simulink model "Flux_Estimator"  (R2014a)
settings: Solver=ode23tb  StartTime=0.0  StopTime=1  MaxStep=50e-6  RelTol=1e-3
libraries: powerlib x10, powerlib_meascontrol x2
settings Model: Creator=ninad gaikawad  LastModifiedBy=ninad gaikawad
settings SolverCC: ZeroCrossControl=EnableAll  ZeroCrossAlgorithm=Adaptive  AutoInsertRateTranBlk=on
settings DebuggingCC: AlgebraicLoopMsg=error

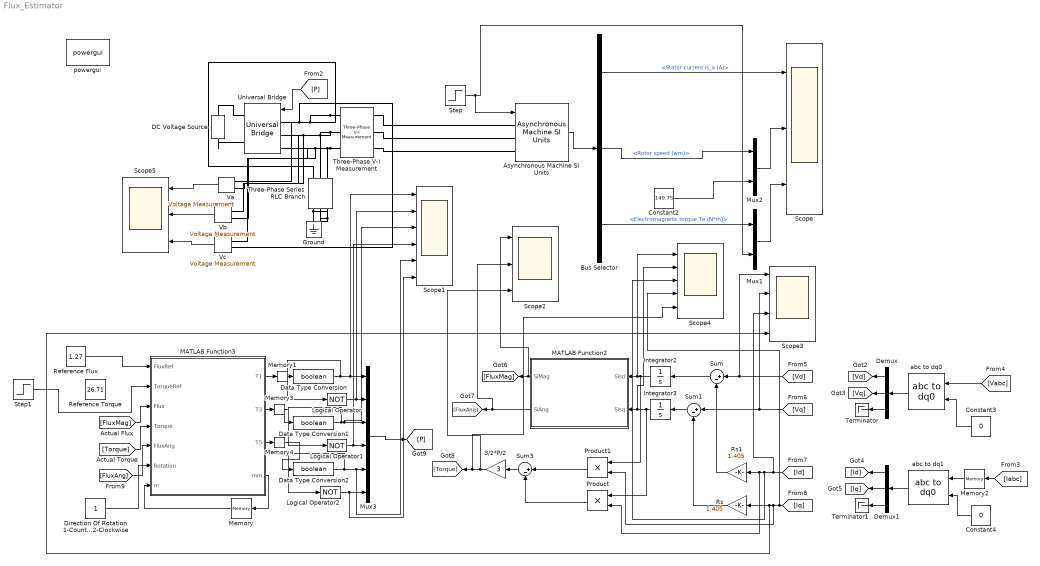
== system Flux_Estimator ==
  3/2*P/2 : Gain  Gain=3
  Asynchronous Machine SI Units : powerlib/Machines/Asynchronous Machine SI Units  PresetModel="15:  5.4 HP (4KW)   400 V  50Hz 1430 RPM"  MechanicalLoad=Torque Tm  ShowDetailedParameters=on  RotorType=Squirrel-cage  ReferenceFrame=Rotor  Units=SI  MeasurementBus=off  NominalParameters=[4000 400 50]  Stator=[1.405 0.005839]  Rotor=[1.395 0.005839]  Cage1=[ 0.022 0.226/377]  Cage2=[ 0.022 0.226/377]  Lm=0.1722  Mechanical=[0.0131 0.002985 2]  PolePairs=2  InitialConditions=[1 0 0 0 0 0 0 0]  SimulateSaturation=off  Saturation=[14.03593122, 27.81365428, 53.79336849, 72.68890987, 97.98006896, 148.6815601, 215.7428561, 302.9841135, 420.4778367 ; 230, 322, 414, 460, 506, 552, 598, 644, 690]  LoadFlowParameters=1492000  TsPowergui=0  TsBlock=-1  IterativeModel=Trapezoidal non iterative  Pmec=0
  Bus Selector : BusSelector  OutputSignals=Stator measurements.Stator current is_a (A),Mechanical.Rotor speed (wm),Mechanical.Electromagnetic torque Te (N*m)
  Constant2 : Constant  Value=149.75
  Constant3 : Constant  Value=0
  Constant4 : Constant  Value=0
  DC Voltage Source : powerlib/Electrical Sources/DC Voltage Source  Amplitude=565.7  Measurements=None
  Data Type Conversion : DataTypeConversion  OutDataTypeStr=boolean
  Data Type Conversion1 : DataTypeConversion  OutDataTypeStr=boolean
  Data Type Conversion2 : DataTypeConversion  OutDataTypeStr=boolean
  Demux : Demux  Outputs=3
  Demux1 : Demux  Outputs=3
  Direction Of Rotation 1-CounterClockwise 2-Clockwise : Constant
  Ground : powerlib/Elements/Ground  LConnTagsString=a
  Integrator2 : Integrator
  Integrator3 : Integrator
  Logical Operator : Logic  Operator=NOT  AllPortsSameDT=off  OutDataTypeStr=boolean
  Logical Operator1 : Logic  Operator=NOT  AllPortsSameDT=off  OutDataTypeStr=boolean
  Logical Operator2 : Logic  Operator=NOT  AllPortsSameDT=off  OutDataTypeStr=boolean
  MATLAB Function2 : MATLAB Function  TreatAsAtomicUnit=on
  MATLAB Function3 : MATLAB Function  TreatAsAtomicUnit=on
  Memory : Memory  X0=1
  Memory1 : Memory  X0=1
  Memory2 : Memory  X0=1
  Memory3 : Memory
  Memory4 : Memory
  Mux1 : Mux  Inputs=2
  Mux2 : Mux  Inputs=2
  Mux3 : Mux  Inputs=6
  Product : Product
  Product1 : Product
  Reference Flux : Constant  Value=1.27
  Reference Torque : Constant  Value=26.71
  Rs : Gain  Gain=1.405
  Rs1 : Gain  Gain=1.405
  Scope : Scope  NumInputPorts=3
      settings: YMin=-0.31398~-350~0  YMax=-0.284078~150~0.00225
  Scope1 : Scope  NumInputPorts=6
      settings: YMin=-5~-5~-5~-5~-5~-5  YMax=5~5~5~5~5~5
  Scope2 : Scope  NumInputPorts=3
      settings: YMin=-5~-5~-5  YMax=5~5~5  SaveName=ScopeData2
  Scope3 : Scope  NumInputPorts=4
      settings: TimeRange=10  YMin=-400~-400~-266.8~-1  YMax=200~400~-266.35~0.5  SaveName=ScopeData3
  Scope4 : Scope  NumInputPorts=5
      settings: YMin=-5~-5~-5~-5~-5  YMax=5~5~5~5~5  SaveName=ScopeData4
  Scope5 : Scope  NumInputPorts=3
      settings: YMin=-5~-5~-5  YMax=5~5~5  SaveName=ScopeData5
  Step : Step  Time=0.5  After=26.71  SampleTime=0
  Step1 : Step  Time=0.5  After=26.71  SampleTime=0
  Sum : Sum  Inputs=|+-
  Sum1 : Sum  Inputs=|+-
  Sum3 : Sum  Inputs=|+-
  Terminator : Terminator
  Terminator1 : Terminator
  Three-Phase Series RLC Branch : powerlib/Elements/Three-Phase Series RLC Branch  LConnTagsString=A|B|C  RConnTagsString=A|B|C  BranchType=R  Resistance=1e6  Inductance=1e-3  Capacitance=1e-6  Measurements=None
  Three-Phase V-I Measurement : powerlib/Measurements/Three-Phase V-I Measurement  VoltageMeasurement=phase-to-ground  SetLabelV=on  LabelV=Vabc  Vpu=off  VpuLL=off  CurrentMeasurement=yes  SetLabelI=on  LabelI=Iabc  Ipu=off  Pbase=100e6  Vbase=500e3  OutputType=Complex  PhasorSimulation=off  PSBequivalent=0
  Universal Bridge : powerlib/Power Electronics/Universal Bridge  Arms=3  SnubberResistance=1e5  SnubberCapacitance=inf  Device=IGBT / Diodes  Ron=1e-3  Lon=0  ForwardVoltages="[  0  0  ]"  ForwardVoltage=0  GTOparameters=[ 10e-6 , 20e-6 ]  IGBTparameters=[ 1e-6 , 2e-6 ]  Measurements=None  Measurements_2=None  converterType=Rectifier
  Va : powerlib/Measurements/Voltage Measurement  PhasorSimulation=off  OutputType=Complex  PSBequivalent=0
  Vb : powerlib/Measurements/Voltage Measurement  PhasorSimulation=off  OutputType=Complex  PSBequivalent=0
  Vc : powerlib/Measurements/Voltage Measurement  PhasorSimulation=off  OutputType=Complex  PSBequivalent=0
  abc to dq0 : powerlib_meascontrol/Transformations/abc to dq0  Alignment=Aligned with phase A axis
  abc to dq1 : powerlib_meascontrol/Transformations/abc to dq0  Alignment=Aligned with phase A axis
  powergui : powerlib/powergui  Priority=1  SimulationMode=Continuous  SolverType=Tustin  SampleTime=50e-6  frequency=60  SPID=off  DisableSnubberDevices=off  DisableRonSwitches=off  DisableVfSwitches=off  SwTol=0  Interpol=off  DisplayEquations=off  Ts=0  methode=off  frequencyindice=50  Pbase=100e6  ErrMax=1e-4  Iterations=50  UnitsV=kV  UnitsW=MW  FunctionMessages=off  echomessages=off  HookPort=off  EnableUseOfTLC=off  x0status=blocks  RestoreLinks=warning  ResistiveCurrentMeasurement=off  Frange=[0:2:500]  Ylog=off  Xlog=on  ShowGrid=off  save=off  variable=ZData  structure=0  ZoomFFT=off  StartTime=0.0  cycles=1  DisplayStyle=1  fundamental=60  FreqAxis=off  MaxFrequency=1000  frequencyindicesteady=1  RmsSteady=1  display=off
  wires:
  Asynchronous Machine SI Units/1 -> Bus Selector/1
  Mux1/1 -> Scope/3
  Mux2/1 -> Scope/2
  [P] -> Universal Bridge/1
  Bus Selector/1 -> Scope/1  "<Stator current is_a (A)>"
  Bus Selector/2 -> Mux2/1  "<Rotor speed (wm)>"
  Bus Selector/3 -> Mux1/1  "<Electromagnetic torque Te (N*m)>"
  Constant2/1 -> Mux2/2
  Constant3/1 -> abc to dq0/2
  Constant4/1 -> abc to dq1/2
  abc to dq0/1 -> Demux/1
  abc to dq1/1 -> Demux1/1
  Demux1/3 -> Terminator1/1
  Demux/3 -> Terminator/1
  Demux1/2 -> [Iq]
  Demux1/1 -> [Id]
  Demux/1 -> [Vd]
  Demux/2 -> [Vq]
  [Id] -> Scope3/3, Scope4/3, Product/2, Rs1/1
  [Iq] -> Scope4/4, Product1/2, Scope3/4, Rs/1
  [Vd] -> Scope3/1, Sum/1
  [Vq] -> Scope3/2, Sum1/1
  Rs1/1 -> Sum/2
  Rs/1 -> Sum1/2
  Sum1/1 -> Integrator3/1
  Sum/1 -> Integrator2/1
  Integrator3/1 -> Product/1, Scope4/2, MATLAB Function2/2(Sisq)
  Integrator2/1 -> Scope4/1, MATLAB Function2/1(Sisd), Product1/1
  Product1/1 -> Sum3/1
  Sum3/1 -> 3/2*P/2/1
  MATLAB Function2/2(SiAng) -> Scope2/2, [FluxAng]
  3/2*P/2/1 -> Scope2/3, Scope4/5, [Torque]
  [FluxAng] -> MATLAB Function3/5(FluxAng)
  [FluxMag] -> MATLAB Function3/3(Flux)
  [Torque] -> MATLAB Function3/4(Torque)
  Reference Flux/1 -> MATLAB Function3/1(FluxRef)
  Direction Of Rotation 1-CounterClockwise 2-Clockwise/1 -> MATLAB Function3/6(Rotation)
  Logical Operator1/1 -> Scope1/4, Mux3/4
  Logical Operator/1 -> Scope1/2, Mux3/2
  Logical Operator2/1 -> Scope1/6, Mux3/6
  Mux3/1 -> [P]
  Data Type Conversion/1 -> Logical Operator/1, Scope1/1, Mux3/1
  Data Type Conversion2/1 -> Logical Operator2/1, Scope1/5, Mux3/5
  Data Type Conversion1/1 -> Logical Operator1/1, Scope1/3, Mux3/3
  MATLAB Function3/4(mm) -> Memory/1
  Memory/1 -> MATLAB Function3/7(m)
  Product/1 -> Sum3/2
  MATLAB Function2/1(SiMag) -> Scope2/1, [FluxMag]
  Step/1 -> Asynchronous Machine SI Units/1, Mux1/2
  [Vabc] -> abc to dq0/1
  Memory2/1 -> abc to dq1/1
  [Iabc] -> Memory2/1
  Memory1/1 -> Data Type Conversion/1
  MATLAB Function3/1(T1) -> Memory1/1
  Memory3/1 -> Data Type Conversion1/1
  MATLAB Function3/2(T3) -> Memory3/1
  MATLAB Function3/3(T5) -> Memory4/1
  Memory4/1 -> Data Type Conversion2/1
  Va/1 -> Scope5/1
  Vb/1 -> Scope5/2
  Vc/1 -> Scope5/3
  Step1/1 -> MATLAB Function3/2(TorqueRef)
  connections:
  Three-Phase V-I Measurement/LConn2 -- Va/LConn2 -- Vb/LConn1 -- Universal Bridge/LConn2 -- Three-Phase Series RLC Branch/LConn2
  Three-Phase V-I Measurement/LConn1 -- Vc/LConn2 -- Va/LConn1 -- Universal Bridge/LConn1 -- Three-Phase Series RLC Branch/LConn1
  Three-Phase V-I Measurement/LConn3 -- Vb/LConn2 -- Vc/LConn1 -- Universal Bridge/LConn3 -- Three-Phase Series RLC Branch/LConn3
  Ground/LConn1 -- Three-Phase Series RLC Branch/RConn3 -- Three-Phase Series RLC Branch/RConn1 -- Three-Phase Series RLC Branch/RConn2
  DC Voltage Source/RConn1 -- Universal Bridge/RConn1
  DC Voltage Source/LConn1 -- Universal Bridge/RConn2
  Asynchronous Machine SI Units/LConn3 -- Three-Phase V-I Measurement/RConn3
  Asynchronous Machine SI Units/LConn2 -- Three-Phase V-I Measurement/RConn2
  Asynchronous Machine SI Units/LConn1 -- Three-Phase V-I Measurement/RConn1

== matlab function Flux_Estimator/MATLAB Function2 ==
  settings: updateMethod=CONTINUOUS
  data: Sisd input; SiMag output; Sisq input; SiAng output
function [SiMag,SiAng] = Flux_Estimator(Sisd,Sisq)
 SiMag=((Sisd)^(2)+(Sisq)^(2))^(0.5);
 x=atan2(Sisq,Sisd);
 if(x>=0)
    SiAng=x*(180/(2*pi));
 else
    SiAng=x*(180/(2*pi))+360;
 end

== matlab function Flux_Estimator/MATLAB Function3 ==
  settings: updateMethod=CONTINUOUS
  data: FluxRef input; TorqueRef input; Flux input; Torque input; T1 output; T3 output; FluxAng input; T5 output; Rotation input; m input; mm output
function [T1,T3,T5,mm] = DTC_SwitchingTable(FluxRef,TorqueRef,Flux,Torque,FluxAng,Rotation,m)
 
T1=0;
T3=0;
T5=0;

DelF=0.0025;% Hysteresis Width for Flux
DelT=0.025;% Hysteresis Width for Torque

Hf=0;%Initializing Hysteresis Controller Output For Flux
Ht=0;%Initializing Hysteresis Controller Output For Torque
S=0;%Initializing DTC Space Vector Sector
mm=m;
% Flux Two Level Hysteresis Band %
%------------------------------------------------------------------------%
if(Flux<=(FluxRef-DelF))
    Hf=1;
    mm=Hf;
end
if(mm==1&&(Flux>(FluxRef-DelF)&&Flux<(FluxRef+DelF)))
    Hf=1;
    mm=Hf;
end
if(Flux>=(FluxRef+DelF))
    Hf=0;
    mm=Hf;
end
if(mm==0&&(Flux>(FluxRef-DelF)&&Flux<(FluxRef+DelF)))
    Hf=0;
    mm=Hf;
end

% Torque Three Level Hysteresis Band %
%------------------------------------------------------------------------%
if(Torque<=(TorqueRef-DelT))
    Ht=1;
end
if(Torque>(TorqueRef-DelT)&&Torque<(TorqueRef+DelT))
    Ht=0;
end
if(Torque>=(TorqueRef+DelT))
    Ht=-1;
end

% DTC Sector Prediction %
%------------------------------------------------------------------------%
if(FluxAng>=330&&FluxAng<30)
    S=1;
end
if(FluxAng>=30&&FluxAng<90)
    S=2;
end
if(FluxAng>=90&&FluxAng<150)
    S=3;
end
if(FluxAng>=150&&FluxAng<210)
    S=4;
end
if(FluxAng>=210&&FluxAng<270)
    S=5;
end
if(FluxAng>=270&&FluxAng<330)
    S=6;
end

% Voltage Vector Synthesis %
%------------------------------------------------------------------------%
if(Rotation==2)% Clockwise Rotation
%------------------------------------------------------------------------%    
    if(Hf==1&&Ht==1&&S==1)
        T1=1;
        T3=0;
        T5=1;
    end
    if(Hf==1&&Ht==1&&S==2)
      T1=0;
      T3=0;
      T5=1;  
    end
    if(Hf==1&&Ht==1&&S==3)
      T1=0;
      T3=1;
      T5=1; 
    end
    if(Hf==1&&Ht==1&&S==4)
      T1=0;
      T3=1;
      T5=0;
    end
    if(Hf==1&&Ht==1&&S==5)
      T1=1;
      T3=1;
      T5=0;    
    end
    if(Hf==1&&Ht==1&&S==6)
      T1=1;
      T3=0;
      T5=0;
    end
   
%------------------------------------------------------------------------%    
    if(Hf==1&&Ht==0&&S==1)
        T1=1;
        T3=1;
        T5=1;
    end
    if(Hf==1&&Ht==0&&S==2)
      T1=0;
      T3=0;
      T5=0;  
    end
    if(Hf==1&&Ht==0&&S==3)
      T1=1;
      T3=1;
      T5=1; 
    end
    if(Hf==1&&Ht==0&&S==4)
      T1=0;
      T3=0;
      T5=0;
    end
    if(Hf==1&&Ht==0&&S==5)
      T1=1;
      T3=1;
      T5=1;    
    end
    if(Hf==1&&Ht==0&&S==6)
      T1=0;
      T3=0;
      T5=0;
    end
%------------------------------------------------------------------------%    
    if(Hf==1&&Ht==-1&&S==1)
        T1=1;
        T3=1;
        T5=0;
    end
    if(Hf==1&&Ht==-1&&S==2)
      T1=1;
      T3=0;
      T5=0;  
    end
    if(Hf==1&&Ht==-1&&S==3)
      T1=1;
      T3=0;
      T5=1; 
    end
    if(Hf==1&&Ht==-1&&S==4)
      T1=0;
      T3=0;
      T5=1;
    end
    if(Hf==1&&Ht==-1&&S==5)
      T1=0;
      T3=1;
      T5=1;    
    end
    if(Hf==1&&Ht==-1&&S==6)
      T1=0;
      T3=1;
      T5=0;
    end
    
 %------------------------------------------------------------------------%   
    
     if(Hf==0&&Ht==1&&S==1)
        T1=0;
        T3=0;
        T5=1;
    end
    if(Hf==0&&Ht==1&&S==2)
      T1=0;
      T3=1;
      T5=1;  
    end
    if(Hf==0&&Ht==1&&S==3)
      T1=0;
      T3=1;
      T5=0; 
    end
    if(Hf==0&&Ht==1&&S==4)
      T1=1;
      T3=1;
      T5=0;
    end
    if(Hf==0&&Ht==1&&S==5)
      T1=1;
      T3=0;
      T5=0;    
    end
    if(Hf==0&&Ht==1&&S==6)
      T1=1;
      T3=0;
      T5=1;
    end
%------------------------------------------------------------------------%    
    
    if(Hf==0&&Ht==0&&S==1)
        T1=0;
        T3=0;
        T5=0;
    end
    if(Hf==0&&Ht==0&&S==2)
      T1=1;
      T3=1;
      T5=1;  
    end
    if(Hf==0&&Ht==0&&S==3)
      T1=0;
      T3=0;
      T5=0; 
    end
    if(Hf==0&&Ht==0&&S==4)
      T1=1;
      T3=1;
      T5=1;
    end
    if(Hf==0&&Ht==0&&S==5)
      T1=0;
      T3=0;
      T5=0;    
    end
    if(Hf==0&&Ht==0&&S==6)
      T1=1;
      T3=1;
      T5=1;
    end
  %------------------------------------------------------------------------%  
    
    if(Hf==0&&Ht==-1&&S==1)
        T1=0;
        T3=1;
        T5=0;
    end
    if(Hf==0&&Ht==-1&&S==2)
      T1=1;
      T3=1;
      T5=0;  
    end
    if(Hf==0&&Ht==-1&&S==3)
      T1=1;
      T3=0;
      T5=0; 
    end
    if(Hf==0&&Ht==-1&&S==4)
      T1=1;
      T3=0;
      T5=1;
    end
    if(Hf==0&&Ht==-1&&S==5)
      T1=0;
      T3=0;
      T5=1;    
    end
    if(Hf==0&&Ht==-1&&S==6)
      T1=0;
      T3=1;
      T5=1;
    end
end

%------------------------------------------------------------------------%
if(Rotation==1)% Counter-Clockwise Rotation
%------------------------------------------------------------------------%    
    if(Hf==1&&Ht==1&&S==1)
        T1=1;
        T3=1;
        T5=0;
    end
    if(Hf==1&&Ht==1&&S==2)
      T1=0;
      T3=1;
      T5=0;  
    end
    if(Hf==1&&Ht==1&&S==3)
      T1=0;
      T3=1;
      T5=1; 
    end
    if(Hf==1&&Ht==1&&S==4)
      T1=0;
      T3=0;
      T5=1;
    end
    if(Hf==1&&Ht==1&&S==5)
      T1=1;
      T3=0;
      T5=1;    
    end
    if(Hf==1&&Ht==1&&S==6)
      T1=1;
      T3=0;
      T5=0;
    end
   
%------------------------------------------------------------------------%    
    if(Hf==1&&Ht==0&&S==1)
        T1=1;
        T3=1;
        T5=1;
    end
    if(Hf==1&&Ht==0&&S==2)
      T1=0;
      T3=0;
      T5=0;  
    end
    if(Hf==1&&Ht==0&&S==3)
      T1=1;
      T3=1;
      T5=1; 
    end
    if(Hf==1&&Ht==0&&S==4)
      T1=0;
      T3=0;
      T5=0;
    end
    if(Hf==1&&Ht==0&&S==5)
      T1=1;
      T3=1;
      T5=1;    
    end
    if(Hf==1&&Ht==0&&S==6)
      T1=0;
      T3=0;
      T5=0;
    end
%------------------------------------------------------------------------%    
    if(Hf==1&&Ht==-1&&S==1)
        T1=1;
        T3=0;
        T5=1;
    end
    if(Hf==1&&Ht==-1&&S==2)
      T1=1;
      T3=0;
      T5=0;  
    end
    if(Hf==1&&Ht==-1&&S==3)
      T1=1;
      T3=1;
      T5=0; 
    end
    if(Hf==1&&Ht==-1&&S==4)
      T1=0;
      T3=1;
      T5=0;
    end
    if(Hf==1&&Ht==-1&&S==5)
      T1=0;
      T3=1;
      T5=1;    
    end
    if(Hf==1&&Ht==-1&&S==6)
      T1=0;
      T3=0;
      T5=1;
    end
    
 %------------------------------------------------------------------------%   
    
     if(Hf==0&&Ht==1&&S==1)
        T1=0;
        T3=1;
        T5=0;
    end
    if(Hf==0&&Ht==1&&S==2)
      T1=0;
      T3=1;
      T5=1;  
    end
    if(Hf==0&&Ht==1&&S==3)
      T1=0;
      T3=0;
      T5=1; 
    end
    if(Hf==0&&Ht==1&&S==4)
      T1=1;
      T3=0;
      T5=1;
    end
    if(Hf==0&&Ht==1&&S==5)
      T1=1;
      T3=0;
      T5=0;    
    end
    if(Hf==0&&Ht==1&&S==6)
      T1=1;
      T3=1;
      T5=0;
    end
%------------------------------------------------------------------------%    
    
    if(Hf==0&&Ht==0&&S==1)
        T1=0;
        T3=0;
        T5=0;
    end
    if(Hf==0&&Ht==0&&S==2)
      T1=1;
      T3=1;
      T5=1;  
    end
    if(Hf==0&&Ht==0&&S==3)
      T1=0;
      T3=0;
      T5=0; 
    end
    if(Hf==0&&Ht==0&&S==4)
      T1=1;
      T3=1;
      T5=1;
    end
    if(Hf==0&&Ht==0&&S==5)
      T1=0;
      T3=0;
      T5=0;    
    end
    if(Hf==0&&Ht==0&&S==6)
      T1=1;
      T3=1;
      T5=1;
    end
  %------------------------------------------------------------------------%  
    
    if(Hf==0&&Ht==-1&&S==1)
        T1=0;
        T3=0;
        T5=1;
    end
    if(Hf==0&&Ht==-1&&S==2)
      T1=1;
      T3=0;
      T5=1;  
    end
    if(Hf==0&&Ht==-1&&S==3)
      T1=1;
      T3=0;
      T5=0; 
    end
    if(Hf==0&&Ht==-1&&S==4)
      T1=1;
      T3=1;
      T5=0;
    end
    if(Hf==0&&Ht==-1&&S==5)
      T1=0;
      T3=1;
      T5=0;    
    end
    if(Hf==0&&Ht==-1&&S==6)
      T1=0;
      T3=1;
      T5=1;
    end
end
